simulink model "rotation_matrix_from_accelerometer"  (R2018a)
settings: Solver=VariableStepAuto  StartTime=0.0  StopTime=10.0  RelTol=1e-3  EnableMultiTasking=on
values from neighbouring files (symbols this model uses):
  aA1 = 10    [init_sim.m]
  aA2 = 0    [init_sim.m]
  aB1 = 0    [init_sim.m]
  aB2 = 0    [init_sim.m]
  aC1 = 0    [init_sim.m]
  aC2 = 0    [init_sim.m]
  gz = 9.810    (= 9.81)    [init_sim.m]
undefined symbols (not defined in the file or in its folder): X, Y, Z
libraries: fl_lib x26, nesl_utility x22, elec_lib x6, sm_lib x4
settings Model: Creator=Asus  LastModifiedBy=Asus
settings DataIOCC: LimitDataPoints=on
settings OptimizationCC: LifeSpan=inf
settings DebuggingCC: AllowSymbolicDim=off  SFUnexpectedBacktrackingDiag=warning  SFNoUnconditionalDefaultTransitionDiag=warning  SFExecutionAtInitializationDiag=none
settings CodeAppCC: StateflowObjectComments=on
settings GRTTargetCC: TargetLangStandard=C89/C90 (ANSI)  GeneratePreprocessorConditionals=Disable all
settings ConfigComp: CovMetricSettings=dw  CovHtmlReporting=on  CovSaveCumulativeToWorkspaceVar=on  CovSaveSingleToWorkspaceVar=on  CovExternalEMLEnable=off  CovSFcnEnable=off
settings SimscapeCC: SimscapeNominalValues="[{\"value\":\"10\",\"unit\":\"V\"},{\"value\":\"1\",\"unit\":\"A\"},{\"value\":\"10\",\"unit\":\"N*m\"},{\"value\":\"10\",\"unit\":\"bar\"},{\"value\":\"100\",\"unit\":\"kJ/kg\"},{\"value\":\"1\",\"unit\":\"kW\"},{\"value\":\"300\",\"unit\":\"K\"},{\"value\":\"100\",\"unit\":\"cm^3/s\"},{\"value\":\"1\",\"unit\":\"kN\"},{\"value\":\"1\",\"unit\":\"g/cm^3\"},{\"value\":\"1\",\"unit\":\"l\"},{\"value\":\"1\",\"unit\":\"cm^2\"},{\"value\":\"60\",\"unit\":\"Hz\"}]"  SimscapeLogType=all  SimscapeLogDataHistory=10000
settings ConfigurationSet: Description=SimMechanics 2G

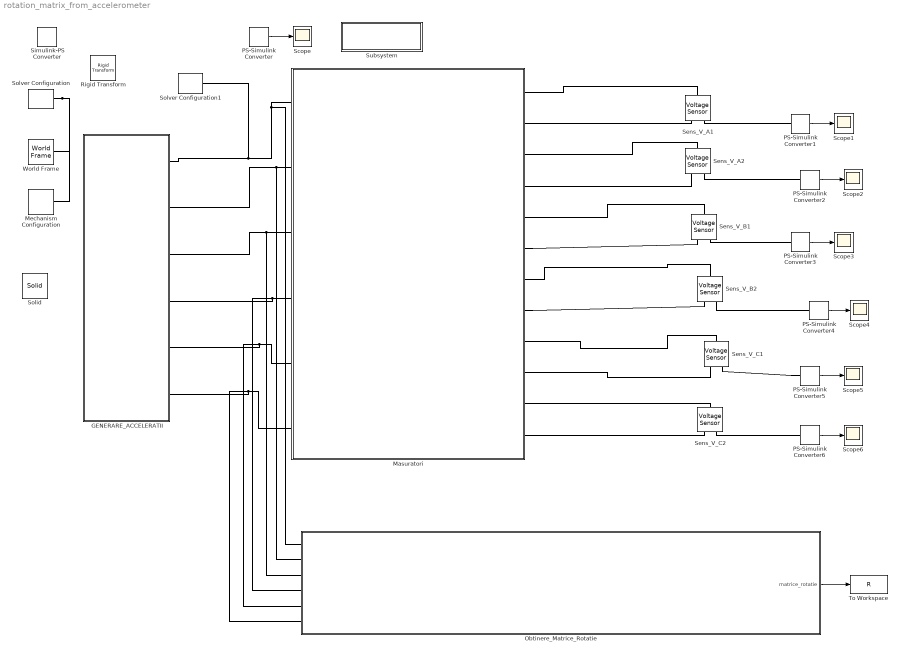
== system rotation_matrix_from_accelerometer ==
  GENERARE_ACCELERATII : Subsystem
  Masuratori : Subsystem
  Mechanism Configuration : sm_lib/Utilities/Mechanism Configuration  UniformGravity=Constant  GravityVector=[0 0 -9.80665]  GravityUnits=m/s^2  LinearizationDelta=0.001
  Obtinere_Matrice_Rotatie : Subsystem
  PS-Simulink Converter{,1..6} (7 alike) : nesl_utility/PS-Simulink Converter  PhysicalDomain=network_engine_domain  SubClassName=ps_output  LeftPortType=input  RightPortType=output  PseudoPeriodic=off  Frequencies=[]  Unit=1  AffineConversion=off
  Rigid Transform : sm_lib/Frames and Transforms/Rigid Transform  TranslationMethod=None  TranslationStandardOffset=0  TranslationLengthUnit=m  TranslationStandardAxis=+Z  TranslationCartesianOffset=[0 0 0]  TranslationROffset=0  TranslationROffsetUnits=m  TranslationZOffset=0  TranslationZOffsetUnits=m  TranslationThetaOffset=0  TranslationThetaOffsetUnits=deg  RotationMethod=None  RotationAngleUnits=deg  RotationStandardAxis=+Z  RotationAngle=0.0  RotationArbitraryAxis=[0 0 1]  FollAlignAxisA=+X  BaseAlignAxisA=+Y  FollAlignAxisB=+Y  BaseAlignAxisB=+Z  RotationSequenceAxes=FollowerAxes  RotationSequence=XYX  RotationSequenceAngles=[0 0 0]  RotationSequenceAnglesUnits=deg  RotationMatrix=[1 0 0; 0 1 0; 0 0 1]
  Scope{,1..6} (7 alike) : Scope
  Sens_V_A1 : fl_lib/Electrical/Electrical Sensors/Voltage Sensor
  Sens_V_A2 : fl_lib/Electrical/Electrical Sensors/Voltage Sensor
  Sens_V_B1 : fl_lib/Electrical/Electrical Sensors/Voltage Sensor
  Sens_V_B2 : fl_lib/Electrical/Electrical Sensors/Voltage Sensor
  Sens_V_C1 : fl_lib/Electrical/Electrical Sensors/Voltage Sensor
  Sens_V_C2 : fl_lib/Electrical/Electrical Sensors/Voltage Sensor
  Simulink-PS Converter : nesl_utility/Simulink-PS Converter  PhysicalDomain=network_engine_domain  SubClassName=ps_input  LeftPortType=input  RightPortType=output  PseudoPeriodic=off  Frequencies=[]  NoiseDistribution=none  NoiseParameters=[]  Unit=1  AffineConversion=off  FilteringAndDerivatives=zero  SimscapeFilterOrder=1  InputFilterTimeConstant=0.001  UdotUserProvided=1
  Solid : sm_lib/Body Elements/Solid  InertiaType=CalculateFromGeometry  Mass=1  MassUnits=kg  CenterOfMass=[0 0 0]  CenterOfMassUnits=m  MomentsOfInertia=[1 1 1]  MomentsOfInertiaUnits=kg*m^2  ProductsOfInertia=[0 0 0]  ProductsOfInertiaUnits=kg*m^2  DensityBased=on  Density=1000  DensityUnits=kg/m^3  DoExposeReferenceFrame=on  SerializedFrames=<Frames/>  GraphicType=FromGeometry  MarkerShape=Sphere  MarkerSize=10  GraphicVisPropType=SimpleVisualProperties  GraphicDiffuseColor=[0.5 0.5 0.5]  GraphicSpecularColor=[0.5 0.5 0.5 1.0]  GraphicAmbientColor=[0.15 0.15 0.15 1.0]  GraphicEmissiveColor=[0.0 0.0 0.0 1.0]  GraphicShininess=75  GraphicOpacity=1.0  GeometryShape=Brick  RectangleSize=[1 1]  RectangleSizeUnits=m  BrickDimensions=[1 1 1]  BrickDimensionUnits=m  CylinderRadius=1  CylinderRadiusUnits=m  CylinderLength=1  CylinderLengthUnits=m  SphereRadius=1  SphereRadiusUnits=m  EllipsoidRadii=[1 1 1]  EllipsoidRadiiUnits=m  ExtrusionCrossSection=[1 1; -1 1; -1 -1; 1 -1]  ExtrusionCrossSectionUnits=m  ExtrusionLength=1  ExtrusionLengthUnits=m  PolygonNumSides=3  PolygonOuterRadius=1  PolygonOuterRadiusUnits=m  ExtGeomFileType=STEP  ExtGeomFileUnits=m  RevolutionCrossSection=[1 1; 1 -1; 2 -1; 2 1]  RevolutionCrossSectionUnits=m  RevolutionExtent=Full  RevolutionAngle=180  RevolutionAngleUnits=deg
  Solver Configuration : nesl_utility/Solver Configuration  PhysicalDomain=network_engine_domain  SubClassName=solver  LeftPortType=input  RightPortType=generic  Tones=[]  Harmonics=[]  SimulateNoise=off  Profile=off  UseLocalSampling=off  EnableSwitchedLinearOptims=on  FrequencyDomain=off  UseCCode=off  RelTol=0.001  AbsTol=1e-06  MinStep=1e-09  ToWorkspace=off  RevertToSquareIcSolve=off  NumHomotopyIterations=100  PhasorMode=off  PhasorModeNumHarmonics=1  DoDC=off  ResidualTolerance=1e-09  UseLocalSolver=off  LocalSolverChoice=NE_BACKWARD_EULER_ADVANCER  LocalSolverSampleTime=0.001  DoFixedCost=off  MaxNonlinIter=3  MaxModeIter=2  LinearAlgebra=Sparse  EquationFormulation=NE_TIME_EF  DelaysMemoryBudget=1024  AutomaticFiltering=on  FilteringTimeConstant=0.001
  Solver Configuration1 : nesl_utility/Solver Configuration  PhysicalDomain=network_engine_domain  SubClassName=solver  LeftPortType=input  RightPortType=generic  Tones=[]  Harmonics=[]  SimulateNoise=off  Profile=off  UseLocalSampling=off  EnableSwitchedLinearOptims=on  FrequencyDomain=off  UseCCode=off  RelTol=0.001  AbsTol=1e-06  MinStep=1e-09  ToWorkspace=off  RevertToSquareIcSolve=off  NumHomotopyIterations=100  PhasorMode=off  PhasorModeNumHarmonics=1  DoDC=off  ResidualTolerance=1e-09  UseLocalSolver=off  LocalSolverChoice=NE_BACKWARD_EULER_ADVANCER  LocalSolverSampleTime=0.001  DoFixedCost=off  MaxNonlinIter=3  MaxModeIter=2  LinearAlgebra=Sparse  EquationFormulation=NE_TIME_EF  DelaysMemoryBudget=1024  AutomaticFiltering=on  FilteringTimeConstant=0.001
  Subsystem : Subsystem
      settings: OpenFcn=open_system('sm_lib')
      mask Display: disp(sprintf('Open Simscape Multibody\nLibrary'));
  To Workspace : ToWorkspace  VariableName=R  SampleTime=-1
  World Frame : sm_lib/Frames and Transforms/World Frame
  wires:
  PS-Simulink Converter/1 -> Scope/1
  PS-Simulink Converter1/1 -> Scope1/1
  PS-Simulink Converter2/1 -> Scope2/1
  PS-Simulink Converter3/1 -> Scope3/1
  PS-Simulink Converter4/1 -> Scope4/1
  PS-Simulink Converter5/1 -> Scope5/1
  PS-Simulink Converter6/1 -> Scope6/1
  Obtinere_Matrice_Rotatie/1(matrice_rotatie) -> To Workspace/1
  connections:
  Solver Configuration/RConn1 -- Mechanism Configuration/RConn1 -- World Frame/RConn1
  PS-Simulink Converter1/LConn1 -- Sens_V_A1/RConn1
  PS-Simulink Converter2/LConn1 -- Sens_V_A2/RConn1
  PS-Simulink Converter3/LConn1 -- Sens_V_B1/RConn1
  Sens_V_B2/RConn1 -- PS-Simulink Converter4/LConn1
  PS-Simulink Converter5/LConn1 -- Sens_V_C1/RConn1
  PS-Simulink Converter6/LConn1 -- Sens_V_C2/RConn1
  Sens_V_A1/LConn1 -- Masuratori/RConn1
  Masuratori/RConn2 -- Sens_V_A1/RConn2
  Masuratori/RConn3 -- Sens_V_A2/LConn1
  GENERARE_ACCELERATII/LConn1 -- Solver Configuration1/RConn1 -- Obtinere_Matrice_Rotatie/LConn1 -- Masuratori/LConn1
  Sens_V_A2/RConn2 -- Masuratori/RConn4
  GENERARE_ACCELERATII/LConn2 -- Obtinere_Matrice_Rotatie/LConn2 -- Masuratori/LConn2
  Masuratori/RConn5 -- Sens_V_B1/LConn1
  Masuratori/RConn6 -- Sens_V_B1/RConn2
  Masuratori/LConn3 -- Obtinere_Matrice_Rotatie/LConn3 -- GENERARE_ACCELERATII/LConn3
  Masuratori/RConn7 -- Sens_V_B2/LConn1
  Masuratori/RConn8 -- Sens_V_B2/RConn2
  Masuratori/LConn4 -- Obtinere_Matrice_Rotatie/LConn4 -- GENERARE_ACCELERATII/LConn4
  Masuratori/RConn9 -- Sens_V_C1/LConn1
  Masuratori/LConn5 -- Obtinere_Matrice_Rotatie/LConn5 -- GENERARE_ACCELERATII/LConn5
  Sens_V_C1/RConn2 -- Masuratori/RConn10
  Masuratori/LConn6 -- Obtinere_Matrice_Rotatie/LConn6 -- GENERARE_ACCELERATII/LConn6
  Masuratori/RConn11 -- Sens_V_C2/LConn1
  Masuratori/RConn12 -- Sens_V_C2/RConn2

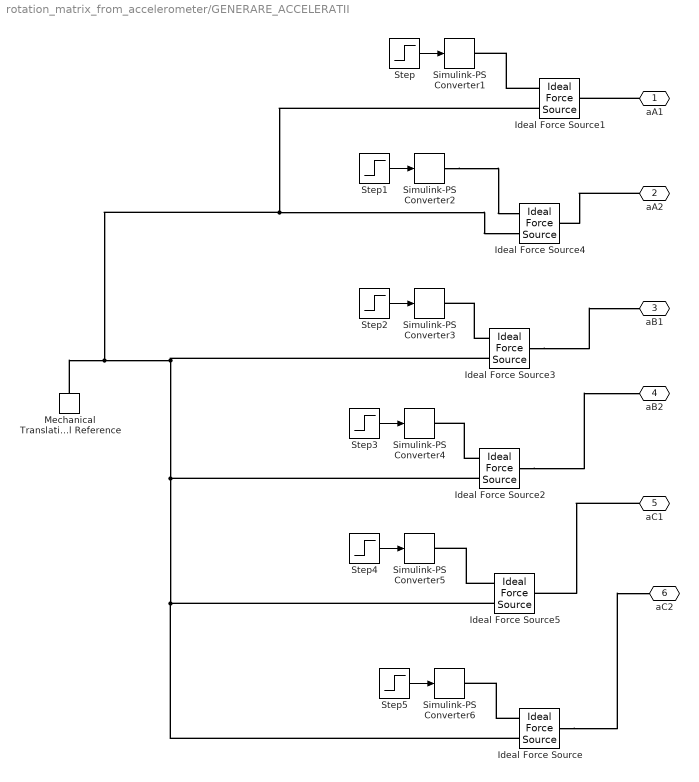
== system rotation_matrix_from_accelerometer/GENERARE_ACCELERATII ==
  Ideal Force Source{,1..5} (6 alike) : fl_lib/Mechanical/Mechanical Sources/Ideal Force Source
  Mechanical Translational Reference : fl_lib/Mechanical/Translational Elements/Mechanical Translational Reference
  Simulink-PS Converter{1..6} (6 alike) : nesl_utility/Simulink-PS Converter  PhysicalDomain=network_engine_domain  SubClassName=ps_input  LeftPortType=input  RightPortType=output  PseudoPeriodic=off  Frequencies=[]  NoiseDistribution=none  NoiseParameters=[]  Unit=1  AffineConversion=off  FilteringAndDerivatives=zero  SimscapeFilterOrder=1  InputFilterTimeConstant=0.001  UdotUserProvided=1
  Step : Step  Time=0.1  After=aA1  SampleTime=0
  Step1 : Step  Time=0.1  After=aA2  SampleTime=0
  Step2 : Step  Time=0.1  After=aB1  SampleTime=0
  Step3 : Step  Time=0.1  After=aB2  SampleTime=0
  Step4 : Step  Time=0.1  After=aC1  SampleTime=0
  Step5 : Step  Time=0.1  After=aC2  SampleTime=0
  aA1 : PMIOPort  Side=Left
  aA2 : PMIOPort  Port=2  Side=Left
  aB1 : PMIOPort  Port=3  Side=Left
  aB2 : PMIOPort  Port=4  Side=Left
  aC1 : PMIOPort  Port=5  Side=Left
  aC2 : PMIOPort  Port=6  Side=Left
  wires:
  Step/1 -> Simulink-PS Converter1/1
  Step3/1 -> Simulink-PS Converter4/1
  Step2/1 -> Simulink-PS Converter3/1
  Step4/1 -> Simulink-PS Converter5/1
  Step1/1 -> Simulink-PS Converter2/1
  Step5/1 -> Simulink-PS Converter6/1
  connections:
  aC1/RConn1 -- Ideal Force Source5/LConn1
  Ideal Force Source2/LConn1 -- aB2/RConn1
  Ideal Force Source1/RConn1 -- Simulink-PS Converter1/RConn1
  Ideal Force Source2/RConn2 -- Ideal Force Source3/RConn2 -- Ideal Force Source4/RConn2 -- Ideal Force Source1/RConn2 -- Mechanical Translational Reference/LConn1 -- Ideal Force Source/RConn2 -- Ideal Force Source5/RConn2
  Ideal Force Source5/RConn1 -- Simulink-PS Converter5/RConn1
  Ideal Force Source2/RConn1 -- Simulink-PS Converter4/RConn1
  Ideal Force Source3/LConn1 -- aB1/RConn1
  Ideal Force Source3/RConn1 -- Simulink-PS Converter3/RConn1
  Ideal Force Source/RConn1 -- Simulink-PS Converter6/RConn1
  Simulink-PS Converter2/RConn1 -- Ideal Force Source4/RConn1
  aA2/RConn1 -- Ideal Force Source4/LConn1
  aA1/RConn1 -- Ideal Force Source1/LConn1
  Ideal Force Source/LConn1 -- aC2/RConn1

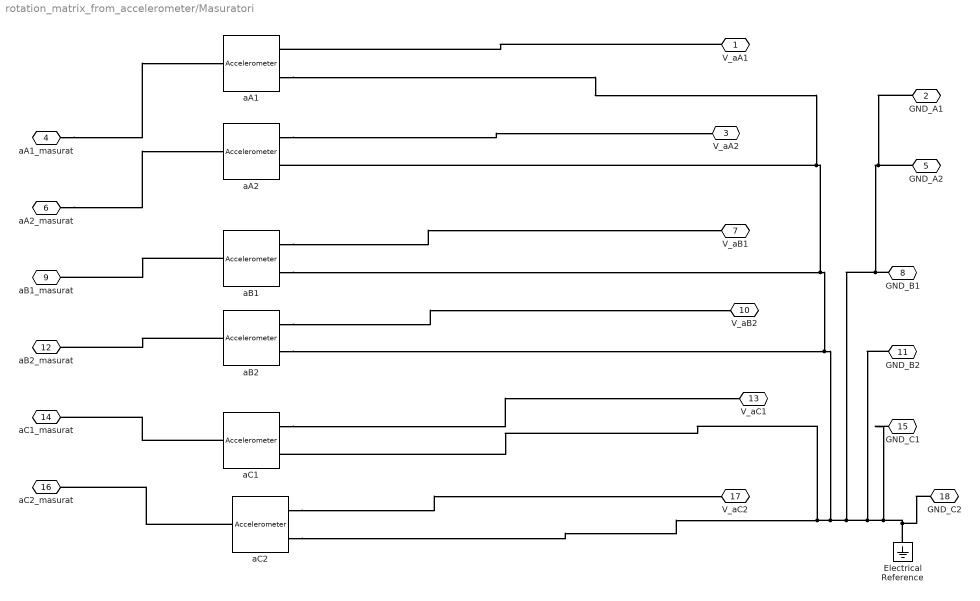
== system rotation_matrix_from_accelerometer/Masuratori ==
  Electrical Reference : fl_lib/Electrical/Electrical Elements/Electrical Reference
  aA1 : elec_lib/Sensors/Accelerometer  output_type=1  sensitivity=1000 mV/gee  sensitivity_pwm=10 1/gee  v_null=2.5 V  duty_cycle0=50  v_max=4 V  duty_cycle_max=75  v_min=1 V  duty_cycle_min=25  F=1000 Hz  Vm=5 V  model_dynamics=0  bw=3 kHz  a_meas_specify=off  a_meas_priority=Low  a_meas=0 m/s^2  a_meas_nominal_specify=off  a_meas_nominal_unit=m/s^2  a_meas_nominal_value=1
      settings: SourceProductName=Simscape Electronics  SourceProductBaseCode=SN
  aA2 : elec_lib/Sensors/Accelerometer  output_type=1  sensitivity=1000 mV/gee  sensitivity_pwm=10 1/gee  v_null=2.5 V  duty_cycle0=50  v_max=4 V  duty_cycle_max=75  v_min=1 V  duty_cycle_min=25  F=1000 Hz  Vm=5 V  model_dynamics=0  bw=3 kHz  a_meas_specify=off  a_meas_priority=Low  a_meas=0 m/s^2  a_meas_nominal_specify=off  a_meas_nominal_unit=m/s^2  a_meas_nominal_value=1
      settings: SourceProductName=Simscape Electronics  SourceProductBaseCode=SN
  aB1 : elec_lib/Sensors/Accelerometer  output_type=1  sensitivity=1000 mV/gee  sensitivity_pwm=10 1/gee  v_null=2.5 V  duty_cycle0=50  v_max=4 V  duty_cycle_max=75  v_min=1 V  duty_cycle_min=25  F=1000 Hz  Vm=5 V  model_dynamics=0  bw=3 kHz  a_meas_specify=off  a_meas_priority=Low  a_meas=0 m/s^2  a_meas_nominal_specify=off  a_meas_nominal_unit=m/s^2  a_meas_nominal_value=1
      settings: SourceProductName=Simscape Electronics  SourceProductBaseCode=SN
  aB2 : elec_lib/Sensors/Accelerometer  output_type=1  sensitivity=1000 mV/gee  sensitivity_pwm=10 1/gee  v_null=2.5 V  duty_cycle0=50  v_max=4 V  duty_cycle_max=75  v_min=1 V  duty_cycle_min=25  F=1000 Hz  Vm=5 V  model_dynamics=0  bw=3 kHz  a_meas_specify=off  a_meas_priority=Low  a_meas=0 m/s^2  a_meas_nominal_specify=off  a_meas_nominal_unit=m/s^2  a_meas_nominal_value=1
      settings: SourceProductName=Simscape Electronics  SourceProductBaseCode=SN
  aC1 : elec_lib/Sensors/Accelerometer  output_type=1  sensitivity=1000 mV/gee  sensitivity_pwm=10 1/gee  v_null=2.5 V  duty_cycle0=50  v_max=4 V  duty_cycle_max=75  v_min=1 V  duty_cycle_min=25  F=1000 Hz  Vm=5 V  model_dynamics=0  bw=3 kHz  a_meas_specify=off  a_meas_priority=Low  a_meas=0 m/s^2  a_meas_nominal_specify=off  a_meas_nominal_unit=m/s^2  a_meas_nominal_value=1
      settings: SourceProductName=Simscape Electronics  SourceProductBaseCode=SN
  aC2 : elec_lib/Sensors/Accelerometer  output_type=1  sensitivity=1e-5 mV/gee  sensitivity_pwm=10 1/gee  v_null=2.5 V  duty_cycle0=50  v_max=5 V  duty_cycle_max=75  v_min=1 V  duty_cycle_min=25  F=1000 Hz  Vm=5 V  model_dynamics=0  bw=3 kHz  a_meas_specify=off  a_meas_priority=Low  a_meas=0 m/s^2  a_meas_nominal_specify=off  a_meas_nominal_unit=m/s^2  a_meas_nominal_value=1
      settings: SourceProductName=Simscape Electronics  SourceProductBaseCode=SN
  V_aA1 : PMIOPort  Side=Right
  GND_A1 : PMIOPort  Port=2  Side=Right
  V_aA2 : PMIOPort  Port=3  Side=Right
  aA1_masurat : PMIOPort  Port=4  Side=Left
  GND_A2 : PMIOPort  Port=5  Side=Right
  aA2_masurat : PMIOPort  Port=6  Side=Left
  V_aB1 : PMIOPort  Port=7  Side=Right
  GND_B1 : PMIOPort  Port=8  Side=Right
  aB1_masurat : PMIOPort  Port=9  Side=Left
  V_aB2 : PMIOPort  Port=10  Side=Right
  GND_B2 : PMIOPort  Port=11  Side=Right
  aB2_masurat : PMIOPort  Port=12  Side=Left
  V_aC1 : PMIOPort  Port=13  Side=Right
  aC1_masurat : PMIOPort  Port=14  Side=Left
  GND_C1 : PMIOPort  Port=15  Side=Right
  aC2_masurat : PMIOPort  Port=16  Side=Left
  V_aC2 : PMIOPort  Port=17  Side=Right
  GND_C2 : PMIOPort  Port=18  Side=Right
  connections:
  aC1/LConn1 -- aC1_masurat/RConn1
  aA2/RConn1 -- V_aA2/RConn1
  aB1/RConn1 -- V_aB1/RConn1
  aB2/RConn1 -- V_aB2/RConn1
  V_aA1/RConn1 -- aA1/RConn1
  aB1/LConn1 -- aB1_masurat/RConn1
  aA2_masurat/RConn1 -- aA2/LConn1
  aC2/RConn1 -- V_aC2/RConn1
  aC1/RConn1 -- V_aC1/RConn1
  aB2/LConn1 -- aB2_masurat/RConn1
  aC2/RConn2 -- aC1/RConn2 -- GND_A1/RConn1 -- GND_A2/RConn1 -- GND_B1/RConn1 -- GND_B2/RConn1 -- GND_C2/RConn1 -- Electrical Reference/LConn1 -- GND_C1/RConn1 -- aA1/RConn2 -- aA2/RConn2 -- aB1/RConn2 -- aB2/RConn2
  aA1_masurat/RConn1 -- aA1/LConn1
  aC2/LConn1 -- aC2_masurat/RConn1

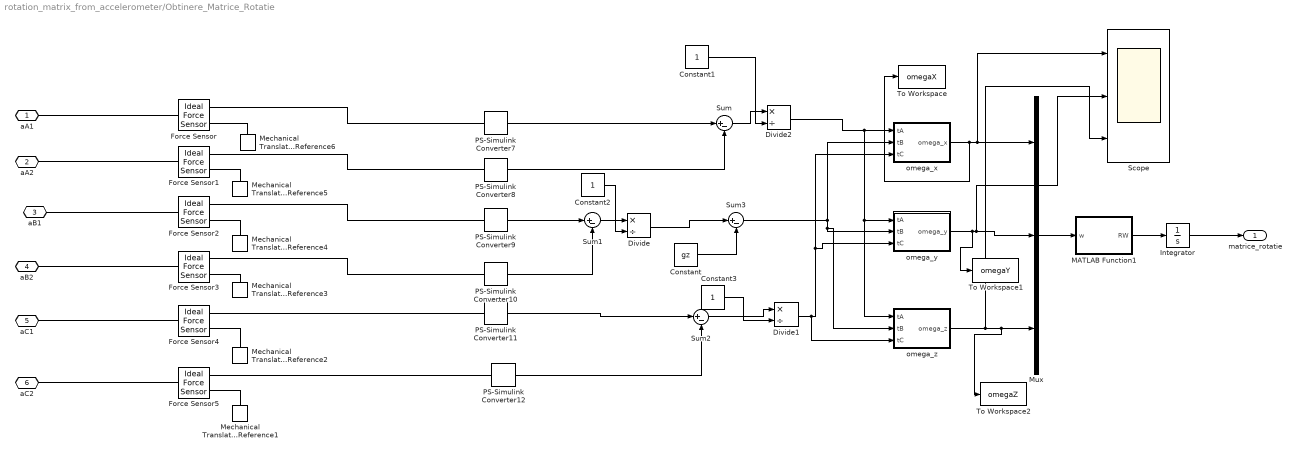
== system rotation_matrix_from_accelerometer/Obtinere_Matrice_Rotatie ==
  Constant : Constant  Value=gz
  Constant1 : Constant
  Constant2 : Constant
  Constant3 : Constant
  Divide : Product  Inputs=*/
  Divide1 : Product  Inputs=*/
  Divide2 : Product  Inputs=*/
  Force Sensor{,1..5} (6 alike) : fl_lib/Mechanical/Mechanical Sensors/Ideal Force Sensor
  Integrator : Integrator
  MATLAB Function1 : MATLAB Function  TreatAsAtomicUnit=on
  Mechanical Translational Reference{1..6} (6 alike) : fl_lib/Mechanical/Translational Elements/Mechanical Translational Reference
  Mux : Mux  Inputs=3
  PS-Simulink Converter{7..12} (6 alike) : nesl_utility/PS-Simulink Converter  PhysicalDomain=network_engine_domain  SubClassName=ps_output  LeftPortType=input  RightPortType=output  PseudoPeriodic=off  Frequencies=[]  Unit=1  AffineConversion=off
  Scope : Scope  NumInputPorts=3
  Sum{,1..3} (4 alike) : Sum  Inputs=|+-
  To Workspace : ToWorkspace  VariableName=omegaX  SaveFormat=Timeseries  SampleTime=-1
  To Workspace1 : ToWorkspace  VariableName=omegaY  SaveFormat=Timeseries  SampleTime=-1
  To Workspace2 : ToWorkspace  VariableName=omegaZ  SaveFormat=Timeseries  SampleTime=-1
  omega_x : MATLAB Function  TreatAsAtomicUnit=on
  omega_y : MATLAB Function  TreatAsAtomicUnit=on
  omega_z : MATLAB Function  TreatAsAtomicUnit=on
  aA1 : PMIOPort  Side=Left
  aA2 : PMIOPort  Port=2  Side=Left
  aB1 : PMIOPort  Port=3  Side=Left
  aB2 : PMIOPort  Port=4  Side=Left
  aC1 : PMIOPort  Port=5  Side=Left
  aC2 : PMIOPort  Port=6  Side=Left
  matrice_rotatie : Outport
  wires:
  Divide1/1 -> omega_z/3(tC), omega_y/3(tC), omega_x/3(tC)
  Sum2/1 -> Divide1/1
  Sum1/1 -> Divide/1
  omega_x/1(omega_x) -> To Workspace/1, Scope/1, Mux/1
  Integrator/1 -> matrice_rotatie/1
  Divide2/1 -> omega_y/1(tA), omega_z/1(tA), omega_x/1(tA)
  omega_y/1(omega_y) -> To Workspace1/1, Scope/2, Mux/2
  MATLAB Function1/1(RW) -> Integrator/1
  Mux/1 -> MATLAB Function1/1(w)
  Sum/1 -> Divide2/1
  PS-Simulink Converter9/1 -> Sum1/1
  PS-Simulink Converter10/1 -> Sum1/2
  Sum3/1 -> omega_z/2(tB), omega_y/2(tB), omega_x/2(tB)
  omega_z/1(omega_z) -> Scope/3, To Workspace2/1, Mux/3
  PS-Simulink Converter7/1 -> Sum/1
  PS-Simulink Converter12/1 -> Sum2/2
  PS-Simulink Converter8/1 -> Sum/2
  PS-Simulink Converter11/1 -> Sum2/1
  Divide/1 -> Sum3/1
  Constant/1 -> Sum3/2
  Constant1/1 -> Divide2/2
  Constant2/1 -> Divide/2
  Constant3/1 -> Divide1/2
  connections:
  Force Sensor5/RConn1 -- Mechanical Translational Reference1/LConn1
  Force Sensor1/RConn2 -- PS-Simulink Converter8/LConn1
  Force Sensor1/LConn1 -- aA2/RConn1
  Force Sensor3/RConn2 -- PS-Simulink Converter10/LConn1
  Mechanical Translational Reference2/LConn1 -- Force Sensor4/RConn1
  Force Sensor3/RConn1 -- Mechanical Translational Reference3/LConn1
  Force Sensor5/LConn1 -- aC2/RConn1
  Mechanical Translational Reference4/LConn1 -- Force Sensor2/RConn1
  PS-Simulink Converter7/LConn1 -- Force Sensor/RConn2
  Mechanical Translational Reference6/LConn1 -- Force Sensor/RConn1
  Force Sensor2/RConn2 -- PS-Simulink Converter9/LConn1
  Mechanical Translational Reference5/LConn1 -- Force Sensor1/RConn1
  Force Sensor/LConn1 -- aA1/RConn1
  Force Sensor4/RConn2 -- PS-Simulink Converter11/LConn1
  PS-Simulink Converter12/LConn1 -- Force Sensor5/RConn2
  Force Sensor3/LConn1 -- aB2/RConn1
  Force Sensor4/LConn1 -- aC1/RConn1
  Force Sensor2/LConn1 -- aB1/RConn1

== system rotation_matrix_from_accelerometer/Subsystem ==

== matlab function rotation_matrix_from_accelerometer/Obtinere_Matrice_Rotatie/omega_y ==
  data: tA input; omega_y output; tB input; tC input
function omega_y  = fcn(tA,tB,tC)

omega_y = 0.5*sign(tC)*sign(tA)*sqrt(abs(tC-tB+tA));

== matlab function rotation_matrix_from_accelerometer/Obtinere_Matrice_Rotatie/omega_x ==
  data: tA input; omega_x output; tB input; tC input
function omega_x = fcn(tA,tB,tC)
    omega_x = 0.5*sign(tB)*sign(tC)*sqrt(abs(tC+tB-tA));

== matlab function rotation_matrix_from_accelerometer/Obtinere_Matrice_Rotatie/omega_z ==
  data: tA input; omega_z output; tB input; tC input
function omega_z = fcn(tA,tB,tC)
omega_z = 0.5*sign(tA)*sign(tB)*sqrt(abs(-tC+tB+tA));

== matlab function rotation_matrix_from_accelerometer/Obtinere_Matrice_Rotatie/MATLAB Function1 ==
  data: w input; RW output
function RW = fcn(w)

RW = zeros(3,3);
RW(1,2) = -w(3);
RW(1,3) = w(2);

RW(2,1) = w(3);
RW(2,3) = -w(1);

RW(3,1) = -w(2);
RW(3,2) = w(1);
